simulink model "Templates"  (R2021a)
settings: Solver=VariableStepAuto  StartTime=0.0  StopTime=10.0  RelTol=1e-3
settings Model: Creator=PC  LastModifiedBy=PC

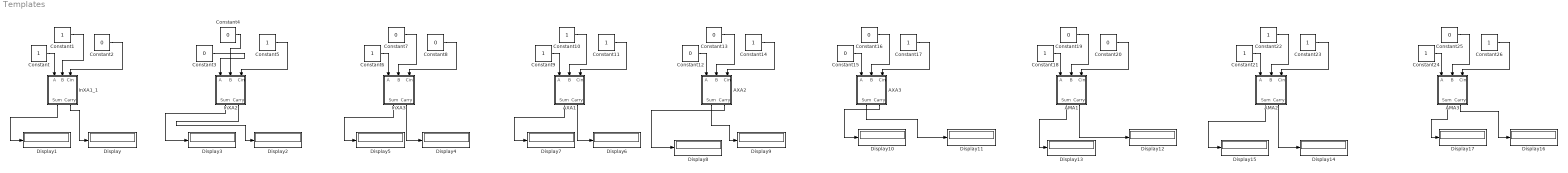
== system Templates ==
  AMA1 : Subsystem
  AMA2 : Subsystem
  AMA3 : Subsystem
  AXA1 : Subsystem
  AXA2 : Subsystem
  AXA3 : Subsystem
  Constant{,1,5..6,9..11,14,17..18,21..24,26} (15 alike) : Constant
  Constant{2..4,7..8,12..13,15..16,19..20,25} (12 alike) : Constant  Value=0
  Display{,1..17} (18 alike) : Display
  InXA1_1 : Subsystem
  InXA2 : Subsystem
  InXA3 : Subsystem
  wires:
  InXA1_1/1(Sum) -> Display1/1
  InXA1_1/2(Carry) -> Display/1
  Constant/1 -> InXA1_1/1(A)
  Constant1/1 -> InXA1_1/2(B)
  Constant2/1 -> InXA1_1/3(Cin)
  Constant3/1 -> InXA2/1(A)
  InXA2/2(Carry) -> Display2/1
  Constant4/1 -> InXA2/2(B)
  Constant5/1 -> InXA2/3(Cin)
  InXA2/1(Sum) -> Display3/1
  Constant6/1 -> InXA3/1(A)
  Constant7/1 -> InXA3/2(B)
  Constant8/1 -> InXA3/3(Cin)
  InXA3/1(Sum) -> Display5/1
  InXA3/2(Carry) -> Display4/1
  AXA1/1(Sum) -> Display7/1
  Constant10/1 -> AXA1/2(B)
  Constant11/1 -> AXA1/3(Cin)
  Constant9/1 -> AXA1/1(A)
  AXA1/2(Carry) -> Display6/1
  AXA2/1(Sum) -> Display9/1
  Constant13/1 -> AXA2/2(B)
  Constant14/1 -> AXA2/3(Cin)
  Constant12/1 -> AXA2/1(A)
  AXA2/2(Carry) -> Display8/1
  Constant15/1 -> AXA3/1(A)
  AXA3/2(Carry) -> Display10/1
  AXA3/1(Sum) -> Display11/1
  Constant16/1 -> AXA3/2(B)
  Constant17/1 -> AXA3/3(Cin)
  Constant20/1 -> AMA1/3(Cin)
  AMA1/1(Sum) -> Display13/1
  Constant18/1 -> AMA1/1(A)
  Constant19/1 -> AMA1/2(B)
  AMA1/2(Carry) -> Display12/1
  Constant21/1 -> AMA2/1(A)
  AMA2/2(Carry) -> Display14/1
  Constant22/1 -> AMA2/2(B)
  Constant23/1 -> AMA2/3(Cin)
  AMA2/1(Sum) -> Display15/1
  Constant24/1 -> AMA3/1(A)
  Constant26/1 -> AMA3/3(Cin)
  Constant25/1 -> AMA3/2(B)
  AMA3/2(Carry) -> Display16/1
  AMA3/1(Sum) -> Display17/1

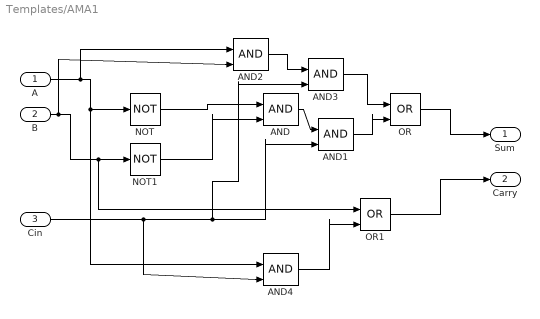
== system Templates/AMA1 ==
  A : Inport
  B : Inport  Port=2
  Cin : Inport  Port=3
  AND{,1..4} (5 alike) : Logic  IconShape=distinctive  AllPortsSameDT=off  OutDataTypeStr=boolean
  NOT : Logic  Operator=NOT  IconShape=distinctive  AllPortsSameDT=off  OutDataTypeStr=boolean
  NOT1 : Logic  Operator=NOT  IconShape=distinctive  AllPortsSameDT=off  OutDataTypeStr=boolean
  OR : Logic  Operator=OR  IconShape=distinctive  AllPortsSameDT=off  OutDataTypeStr=boolean
  OR1 : Logic  Operator=OR  IconShape=distinctive  AllPortsSameDT=off  OutDataTypeStr=boolean
  Sum : Outport
  Carry : Outport  Port=2
  wires:
  A/1 -> AND2/1, AND4/1, NOT/1
  B/1 -> AND2/2, NOT1/1, OR1/1
  NOT/1 -> AND/1
  NOT1/1 -> AND/2
  AND/1 -> AND1/1
  Cin/1 -> AND4/2, AND3/2, AND1/2
  AND2/1 -> AND3/1
  AND3/1 -> OR/1
  AND1/1 -> OR/2
  OR/1 -> Sum/1
  AND4/1 -> OR1/2
  OR1/1 -> Carry/1

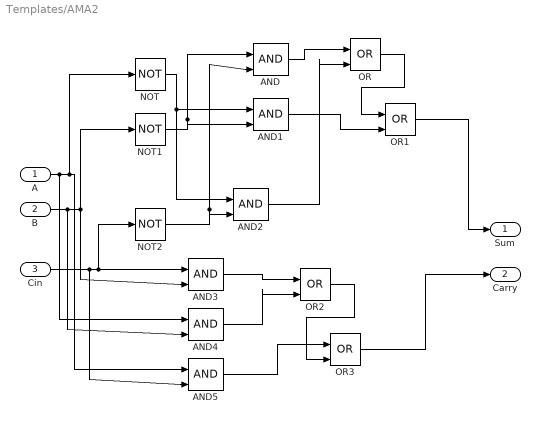
== system Templates/AMA2 ==
  A : Inport
  B : Inport  Port=2
  Cin : Inport  Port=3
  AND{,1..5} (6 alike) : Logic  IconShape=distinctive  AllPortsSameDT=off  OutDataTypeStr=boolean
  NOT : Logic  Operator=NOT  IconShape=distinctive  AllPortsSameDT=off  OutDataTypeStr=boolean
  NOT1 : Logic  Operator=NOT  IconShape=distinctive  AllPortsSameDT=off  OutDataTypeStr=boolean
  NOT2 : Logic  Operator=NOT  IconShape=distinctive  AllPortsSameDT=off  OutDataTypeStr=boolean
  OR{,1..3} (4 alike) : Logic  Operator=OR  IconShape=distinctive  AllPortsSameDT=off  OutDataTypeStr=boolean
  Sum : Outport
  Carry : Outport  Port=2
  wires:
  A/1 -> AND4/1, AND5/1, NOT/1
  B/1 -> AND4/2, AND3/2, NOT1/1
  Cin/1 -> AND5/2, AND3/1, NOT2/1
  NOT2/1 -> AND2/2, AND/2
  NOT1/1 -> AND1/2, AND/1
  NOT/1 -> AND2/1, AND1/1
  AND2/1 -> OR/2
  AND/1 -> OR/1
  OR/1 -> OR1/1
  AND1/1 -> OR1/2
  OR1/1 -> Sum/1
  AND3/1 -> OR2/1
  AND4/1 -> OR2/2
  AND5/1 -> OR3/1
  OR2/1 -> OR3/2
  OR3/1 -> Carry/1

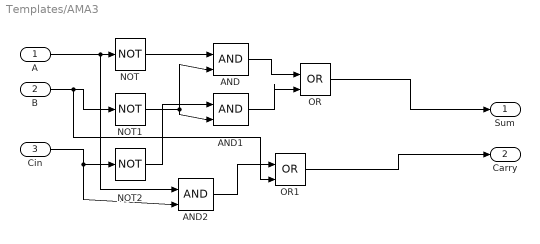
== system Templates/AMA3 ==
  A : Inport
  B : Inport  Port=2
  Cin : Inport  Port=3
  AND : Logic  IconShape=distinctive  AllPortsSameDT=off  OutDataTypeStr=boolean
  AND1 : Logic  IconShape=distinctive  AllPortsSameDT=off  OutDataTypeStr=boolean
  AND2 : Logic  IconShape=distinctive  AllPortsSameDT=off  OutDataTypeStr=boolean
  NOT : Logic  Operator=NOT  IconShape=distinctive  AllPortsSameDT=off  OutDataTypeStr=boolean
  NOT1 : Logic  Operator=NOT  IconShape=distinctive  AllPortsSameDT=off  OutDataTypeStr=boolean
  NOT2 : Logic  Operator=NOT  IconShape=distinctive  AllPortsSameDT=off  OutDataTypeStr=boolean
  OR : Logic  Operator=OR  IconShape=distinctive  AllPortsSameDT=off  OutDataTypeStr=boolean
  OR1 : Logic  Operator=OR  IconShape=distinctive  AllPortsSameDT=off  OutDataTypeStr=boolean
  Sum : Outport
  Carry : Outport  Port=2
  wires:
  A/1 -> AND2/1, NOT/1
  B/1 -> OR1/2, NOT1/1
  NOT/1 -> AND/1
  NOT1/1 -> AND1/2, AND/2
  Cin/1 -> AND2/2, NOT2/1
  NOT2/1 -> AND1/1
  AND/1 -> OR/1
  AND1/1 -> OR/2
  OR/1 -> Sum/1
  AND2/1 -> OR1/1
  OR1/1 -> Carry/1

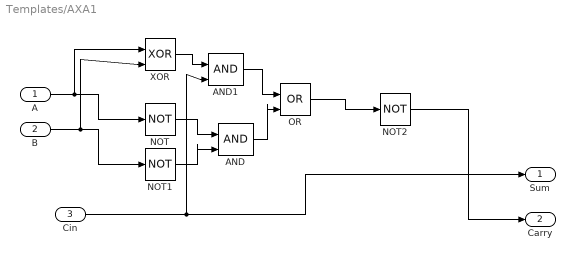
== system Templates/AXA1 ==
  A : Inport
  B : Inport  Port=2
  Cin : Inport  Port=3
  AND : Logic  IconShape=distinctive  AllPortsSameDT=off  OutDataTypeStr=boolean
  AND1 : Logic  IconShape=distinctive  AllPortsSameDT=off  OutDataTypeStr=boolean
  NOT : Logic  Operator=NOT  IconShape=distinctive  AllPortsSameDT=off  OutDataTypeStr=boolean
  NOT1 : Logic  Operator=NOT  IconShape=distinctive  AllPortsSameDT=off  OutDataTypeStr=boolean
  NOT2 : Logic  Operator=NOT  IconShape=distinctive  AllPortsSameDT=off  OutDataTypeStr=boolean
  OR : Logic  Operator=OR  IconShape=distinctive  AllPortsSameDT=off  OutDataTypeStr=boolean
  XOR : Logic  Operator=XOR  IconShape=distinctive  AllPortsSameDT=off  OutDataTypeStr=boolean
  Sum : Outport
  Carry : Outport  Port=2
  wires:
  Cin/1 -> Sum/1, AND1/2
  A/1 -> XOR/1, NOT/1
  B/1 -> XOR/2, NOT1/1
  NOT/1 -> AND/1
  NOT1/1 -> AND/2
  XOR/1 -> AND1/1
  AND1/1 -> OR/1
  AND/1 -> OR/2
  OR/1 -> NOT2/1
  NOT2/1 -> Carry/1

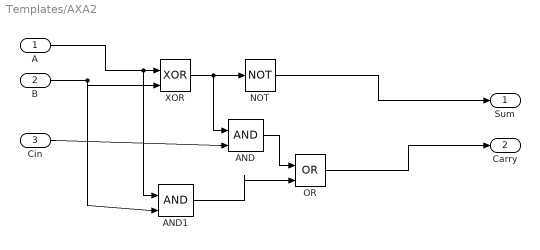
== system Templates/AXA2 ==
  A : Inport
  B : Inport  Port=2
  Cin : Inport  Port=3
  AND : Logic  IconShape=distinctive  AllPortsSameDT=off  OutDataTypeStr=boolean
  AND1 : Logic  IconShape=distinctive  AllPortsSameDT=off  OutDataTypeStr=boolean
  NOT : Logic  Operator=NOT  IconShape=distinctive  AllPortsSameDT=off  OutDataTypeStr=boolean
  OR : Logic  Operator=OR  IconShape=distinctive  AllPortsSameDT=off  OutDataTypeStr=boolean
  XOR : Logic  Operator=XOR  IconShape=distinctive  AllPortsSameDT=off  OutDataTypeStr=boolean
  Sum : Outport
  Carry : Outport  Port=2
  wires:
  NOT/1 -> Sum/1
  A/1 -> AND1/1, XOR/1
  B/1 -> AND1/2, XOR/2
  XOR/1 -> AND/1, NOT/1
  Cin/1 -> AND/2
  AND/1 -> OR/1
  AND1/1 -> OR/2
  OR/1 -> Carry/1

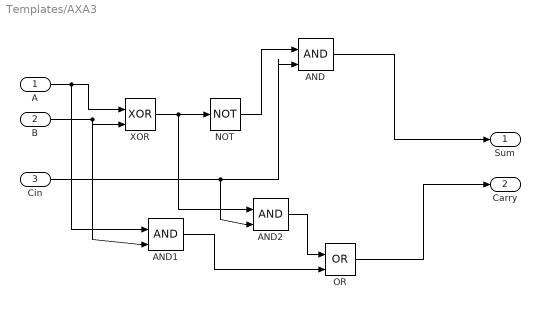
== system Templates/AXA3 ==
  A : Inport
  B : Inport  Port=2
  Cin : Inport  Port=3
  AND : Logic  IconShape=distinctive  AllPortsSameDT=off  OutDataTypeStr=boolean
  AND1 : Logic  IconShape=distinctive  AllPortsSameDT=off  OutDataTypeStr=boolean
  AND2 : Logic  IconShape=distinctive  AllPortsSameDT=off  OutDataTypeStr=boolean
  NOT : Logic  Operator=NOT  IconShape=distinctive  AllPortsSameDT=off  OutDataTypeStr=boolean
  OR : Logic  Operator=OR  IconShape=distinctive  AllPortsSameDT=off  OutDataTypeStr=boolean
  XOR : Logic  Operator=XOR  IconShape=distinctive  AllPortsSameDT=off  OutDataTypeStr=boolean
  Sum : Outport
  Carry : Outport  Port=2
  wires:
  AND/1 -> Sum/1
  B/1 -> XOR/2, AND1/2
  A/1 -> AND1/1, XOR/1
  XOR/1 -> AND2/1, NOT/1
  Cin/1 -> AND2/2, AND/2
  NOT/1 -> AND/1
  AND1/1 -> OR/2
  AND2/1 -> OR/1
  OR/1 -> Carry/1

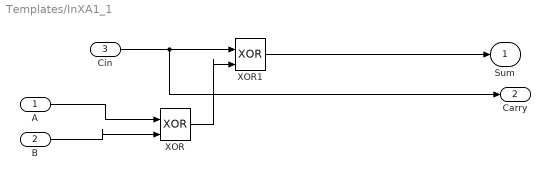
== system Templates/InXA1_1 ==
  A : Inport
  B : Inport  Port=2
  Cin : Inport  Port=3
  XOR : Logic  Operator=XOR  IconShape=distinctive  AllPortsSameDT=off  OutDataTypeStr=boolean
  XOR1 : Logic  Operator=XOR  IconShape=distinctive  AllPortsSameDT=off  OutDataTypeStr=boolean
  Sum : Outport
  Carry : Outport  Port=2
  wires:
  Cin/1 -> Carry/1, XOR1/1
  XOR1/1 -> Sum/1
  A/1 -> XOR/1
  B/1 -> XOR/2
  XOR/1 -> XOR1/2

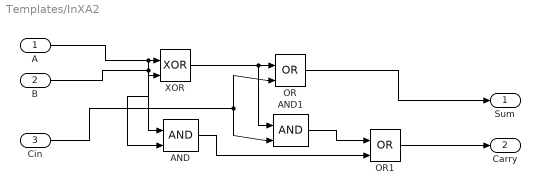
== system Templates/InXA2 ==
  A : Inport
  B : Inport  Port=2
  Cin : Inport  Port=3
  AND : Logic  IconShape=distinctive  AllPortsSameDT=off  OutDataTypeStr=boolean
  AND1 : Logic  IconShape=distinctive  AllPortsSameDT=off  OutDataTypeStr=boolean
  OR : Logic  Operator=OR  IconShape=distinctive  AllPortsSameDT=off  OutDataTypeStr=boolean
  OR1 : Logic  Operator=OR  IconShape=distinctive  AllPortsSameDT=off  OutDataTypeStr=boolean
  XOR : Logic  Operator=XOR  IconShape=distinctive  AllPortsSameDT=off  OutDataTypeStr=boolean
  Sum : Outport
  Carry : Outport  Port=2
  wires:
  A/1 -> AND/1, XOR/1
  B/1 -> AND/2, XOR/2
  Cin/1 -> AND1/2, OR/2
  XOR/1 -> AND1/1, OR/1
  AND1/1 -> OR1/1
  AND/1 -> OR1/2
  OR1/1 -> Carry/1
  OR/1 -> Sum/1

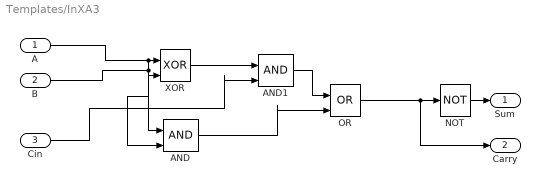
== system Templates/InXA3 ==
  A : Inport
  B : Inport  Port=2
  Cin : Inport  Port=3
  AND : Logic  IconShape=distinctive  AllPortsSameDT=off  OutDataTypeStr=boolean
  AND1 : Logic  IconShape=distinctive  AllPortsSameDT=off  OutDataTypeStr=boolean
  NOT : Logic  Operator=NOT  IconShape=distinctive  AllPortsSameDT=off  OutDataTypeStr=boolean
  OR : Logic  Operator=OR  IconShape=distinctive  AllPortsSameDT=off  OutDataTypeStr=boolean
  XOR : Logic  Operator=XOR  IconShape=distinctive  AllPortsSameDT=off  OutDataTypeStr=boolean
  Sum : Outport
  Carry : Outport  Port=2
  wires:
  A/1 -> AND/1, XOR/1
  B/1 -> AND/2, XOR/2
  Cin/1 -> AND1/2
  XOR/1 -> AND1/1
  AND/1 -> OR/2
  AND1/1 -> OR/1
  OR/1 -> NOT/1, Carry/1
  NOT/1 -> Sum/1
